simulink model "DC_5L"  (R2017b)
settings: Solver=VariableStepAuto  StartTime=0.0  StopTime=2  MaxStep=1e-4  RelTol=1e-3
libraries: powerlib x69, peTransforms x1, powerlib_meascontrol x1
settings Model: Creator=alfonso  LastModifiedBy=alfonso

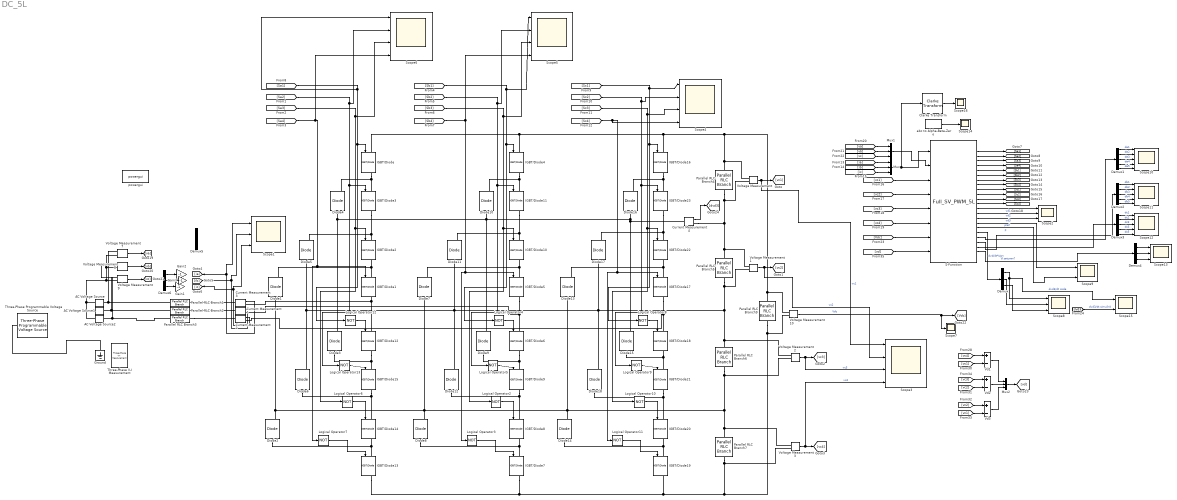
== system DC_5L ==
  AC Voltage Source : powerlib/Electrical Sources/AC Voltage Source  Amplitude=230*sqrt(2)  Phase=0  Frequency=50  SampleTime=0  Measurements=None  BusType=swing  Pref=10e3  Qref=0  Qmin=-inf  Qmax=+inf
  AC Voltage Source1 : powerlib/Electrical Sources/AC Voltage Source  Amplitude=230*sqrt(2)  Phase=120  Frequency=50  SampleTime=0  Measurements=None  BusType=swing  Pref=10e3  Qref=0  Qmin=-inf  Qmax=+inf
  AC Voltage Source2 : powerlib/Electrical Sources/AC Voltage Source  Amplitude=230*sqrt(2)  Phase=240  Frequency=50  SampleTime=0  Measurements=None  BusType=swing  Pref=10e3  Qref=0  Qmin=-inf  Qmax=+inf
  Clarke Transform : peTransforms/Clarke Transform  PowerInvariant=on
  Current Measurement{1..4} (4 alike) : powerlib/Measurements/Current Measurement  PhasorSimulation=off  OutputType=Complex  PSBequivalent=0
  Demux{,4..6} (4 alike) : Demux  Outputs=3
  Demux1 : Demux  Outputs=5
  Demux2 : Demux  Outputs=5
  Demux3 : Demux  Outputs=5
  Diode{1..18} (18 alike) : powerlib/Power Electronics/Diode  Ron=0.001  Lon=0  Vf=0.8  IC=0  UseSnubber=0  Rs=500  Cs=250e-9  Measurements=on
  Gain1 : Gain  Gain=-1
  Gain2 : Gain  Gain=-1
  Gain3 : Gain  Gain=-1
  Ground : powerlib/Elements/Ground  LConnTagsString=a
  IGBT/Diode{,1..23} (24 alike) : powerlib/Power Electronics/IGBT//Diode  Ron=1e-3  Rs=1e5  Cs=inf  Measurements=on
  Logical Operator{2..13} (12 alike) : Logic  Operator=NOT  AllPortsSameDT=off  OutDataTypeStr=boolean
  Mux : Mux  Inputs=3
  Mux1 : Mux  Inputs=3
  Mux2 : Mux  Inputs=3
  Parallel RLC Branch1 : powerlib/Elements/Parallel RLC Branch  LConnTagsString=a  RConnTagsString=__new0  BranchType=L  Resistance=0  Inductance=2e-3  SetiL0=off  InitialCurrent=0  Capacitance=7e-3  Setx0=off  InitialVoltage=0  Measurements=None
  Parallel RLC Branch2 : powerlib/Elements/Parallel RLC Branch  LConnTagsString=a  RConnTagsString=__new0  BranchType=L  Resistance=0  Inductance=2e-3  SetiL0=off  InitialCurrent=0  Capacitance=7e-3  Setx0=off  InitialVoltage=0  Measurements=None
  Parallel RLC Branch3 : powerlib/Elements/Parallel RLC Branch  LConnTagsString=a  RConnTagsString=__new0  BranchType=L  Resistance=0  Inductance=2e-3  SetiL0=off  InitialCurrent=0  Capacitance=7e-3  Setx0=off  InitialVoltage=0  Measurements=None
  Parallel RLC Branch{4..7} (4 alike) : powerlib/Elements/Parallel RLC Branch  LConnTagsString=a  RConnTagsString=__new0  BranchType=C  Resistance=0  Inductance=0  SetiL0=off  InitialCurrent=0  Capacitance=3.3e-3  Setx0=off  InitialVoltage=0  Measurements=None
  Parallel RLC Branch9 : powerlib/Elements/Parallel RLC Branch  LConnTagsString=a  RConnTagsString=__new0  BranchType=R  Resistance=300  Inductance=0  SetiL0=off  InitialCurrent=0  Capacitance=1e-3  Setx0=off  InitialVoltage=0  Measurements=None
  S-Function : S-Function  FunctionName=Full_SV_PWM_5L  SFunctionDeploymentMode=off  EnableBusSupport=off
  Scope{1..2,8,13} (4 alike) : Scope  NumInputPorts=3
  Scope10 : Scope  NumInputPorts=5
  Scope11 : Scope  NumInputPorts=5
  Scope12 : Scope  NumInputPorts=5
  Scope14 : Scope
  Scope15 : Scope  NumInputPorts=2
  Scope16 : Scope
  Scope{3..6} (4 alike) : Scope  NumInputPorts=4
  Scope7 : Scope
  Scope9 : Scope  NumInputPorts=2
  Three-Phase Programmable Voltage Source : powerlib/Electrical Sources/Three-Phase Programmable Voltage Source  PositiveSequence="[230*sqrt(3)  0 50]"  VariationEntity=None  VariationType=Table of time-amplitude pairs  VariationTypeAlt=Step  VariationStep=0.5  VariationRate=10  VariationMagnitude=0.3  VariationFrequency=2  VariationTiming=[1 2]  VariationPhaseA=off  Amplitudes=[1 0.8 1.2 1.0]  TimeValues=[0 0.1 0.15 0.2]  HarmonicGeneration=off  HarmonicA=[3 0.2 -25 0]  HarmonicB=[2 0.15 35 2]  Timing="[0.05  3]"  BusType=swing  Pref=0  Qref=0  Qmin=-inf  Qmax=inf
  Three-Phase V-I Measurement : powerlib/Measurements/Three-Phase V-I Measurement  VoltageMeasurement=phase-to-ground  SetLabelV=off  LabelV=Vabc  Vpu=off  VpuLL=off  CurrentMeasurement=yes  SetLabelI=off  LabelI=Iabc  Ipu=off  Pbase=100e6  Vbase=500e3  OutputType=Complex  PhasorSimulation=off  PSBequivalent=0
  Vd1 : Sum  Inputs=+-
  Vd2 : Sum  Inputs=+-
  Vd3 : Sum  Inputs=+-
  Voltage Measurement{,1..3,7..10} (8 alike) : powerlib/Measurements/Voltage Measurement  PhasorSimulation=off  OutputType=Complex  PSBequivalent=0
  abc to Alpha-Beta-Zero : powerlib_meascontrol/Transformations/abc to Alpha-Beta-Zero
      settings: SourceProductName=Simscape Power Systems
  powergui : powerlib/powergui  Priority=1  SimulationMode=Continuous  SampleTime=50e-6  frequency=60  Iterations=50  frequencyindice=50  Pbase=100e6  ErrMax=1e-4  UnitsV=kV  UnitsW=MW  buscounter=0  FunctionMessages=off  echomessages=off  EnableUseOfTLC=off  CurrentSourceSwitches=off  DisableSnubberDevices=off  DisableRonSwitches=off  DisableVfSwitches=off  DisplayEquations=off  SolverType=Tustin/Backward Euler (TBE)  Interpol=off  ExternalGateDelay=off  methode=off  Ts=100  x0status=blocks  SPID=on  SwTol=0  HookPort=off  RestoreLinks=warning  ResistiveCurrentMeasurement=off  Frange=[0:2:500]  Ylog=off  Xlog=on  ShowGrid=off  save=off  variable=ZData  structure=0  ZoomFFT=off  StartTime=0.0  cycles=1  DisplayStyle=1  fundamental=60  FreqAxis=off  MaxFrequency=1000  frequencyindicesteady=1  RmsSteady=1  display=off
  wires:
  [Sc2] -> Scope4/2, IGBT/Diode23/1, Logical Operator9/1
  [Sc3] -> Scope4/3, Logical Operator10/1, IGBT/Diode22/1
  [Sc4] -> Scope4/4, IGBT/Diode17/1, Logical Operator11/1
  Logical Operator11/1 -> IGBT/Diode19/1
  Logical Operator10/1 -> IGBT/Diode20/1
  Logical Operator9/1 -> IGBT/Diode21/1
  Logical Operator8/1 -> IGBT/Diode18/1
  Logical Operator3/1 -> IGBT/Diode7/1
  Logical Operator4/1 -> IGBT/Diode6/1
  Logical Operator5/1 -> IGBT/Diode9/1
  Logical Operator2/1 -> IGBT/Diode8/1
  Logical Operator6/1 -> IGBT/Diode14/1
  Logical Operator7/1 -> IGBT/Diode13/1
  Logical Operator13/1 -> IGBT/Diode15/1
  Logical Operator12/1 -> IGBT/Diode12/1
  Voltage Measurement/1 -> Scope3/1, [vc1]  "vc1"
  Voltage Measurement1/1 -> Scope3/2, [vc2]  "vc2"
  Voltage Measurement2/1 -> Scope3/3, [vc3]  "vc3"
  Voltage Measurement3/1 -> Scope3/4, [vc4]  "vc4"
  [ia] -> Mux/1
  [ib] -> Mux/2
  [ic] -> Mux/3
  S-Function/12 -> [Sc4]
  S-Function/11 -> [Sc3]
  S-Function/10 -> [Sc2]
  S-Function/9 -> [Sc1]
  S-Function/8 -> [Sb4]
  S-Function/7 -> [Sb3]
  S-Function/6 -> [Sb2]
  S-Function/5 -> [Sb1]
  S-Function/4 -> [Sa4]
  S-Function/1 -> [Sa1]
  S-Function/2 -> [Sa2]
  S-Function/3 -> [Sa3]
  S-Function/13 -> Scope2/1  "vd1"
  S-Function/14 -> Scope2/2  "vd2"
  S-Function/15 -> Scope2/3  "vd3"
  [Sc1] -> Scope4/1, IGBT/Diode16/1, Logical Operator8/1
  S-Function/16 -> Scope9/1  "pref"
  [vc4] -> S-Function/6
  [vc3] -> S-Function/5
  [vc2] -> S-Function/4
  [vc1] -> S-Function/3
  [vc] -> Mux1/3
  [vb] -> Mux1/2
  [va] -> Mux1/1
  [Sb2] -> Scope5/2, IGBT/Diode11/1, Logical Operator5/1
  [Sb3] -> Scope5/3, IGBT/Diode10/1, Logical Operator2/1
  [Sb1] -> Scope5/1, IGBT/Diode4/1, Logical Operator4/1
  [Sb4] -> Logical Operator3/1, IGBT/Diode5/1, Scope5/4
  [Sa3] -> Scope6/3, IGBT/Diode2/1, Logical Operator6/1
  [Sa2] -> Scope6/2, IGBT/Diode3/1, Logical Operator13/1
  [Sa4] -> Scope6/4, Logical Operator7/1, IGBT/Diode1/1
  [Sa1] -> Scope6/1, IGBT/Diode/1, Logical Operator12/1
  Voltage Measurement10/1 -> Scope7/1, [Vdc]  "Vdc"
  Current Measurement3/1 -> [ia], Scope1/1
  Current Measurement2/1 -> [ic], Scope1/3
  [Vdc] -> S-Function/7
  Mux1/1 -> S-Function/2
  S-Function/17 -> Scope9/2  "p"
  S-Function/18 -> Demux/1  "dvd/dt*sign"
  Demux/1 -> Scope15/1, Scope8/1  "dvd3/dt code"
  Demux/2 -> Scope8/2
  Demux/3 -> Scope8/3
  S-Function/22 -> Demux4/1  "d saturan?"
  S-Function/21 -> Demux3/1
  S-Function/20 -> Demux2/1
  S-Function/19 -> Demux1/1
  Demux1/1 -> Scope10/1  "da1"
  Demux1/2 -> Scope10/2  "da2"
  Demux1/3 -> Scope10/3  "da3"
  Demux1/4 -> Scope10/4  "da4"
  Demux2/4 -> Scope11/4  "db4"
  Demux2/2 -> Scope11/2  "db2"
  Demux2/3 -> Scope11/3  "db3"
  Demux2/1 -> Scope11/1  "db1"
  Demux3/4 -> Scope12/4  "dc3"
  Demux3/2 -> Scope12/2  "dc2"
  Demux3/3 -> Scope12/3  "dc3"
  Demux3/1 -> Scope12/1  "dc1"
  Demux4/1 -> Scope13/1
  Demux4/2 -> Scope13/2
  Demux4/3 -> Scope13/3
  Demux3/5 -> Scope12/5  "dc5"
  Demux2/5 -> Scope11/5  "db5"
  Demux1/5 -> Scope10/5  "da5"
  Demux6/1 -> Gain2/1
  Demux6/2 -> Gain3/1
  Demux6/3 -> Gain1/1
  Current Measurement1/1 -> [ib], Scope1/2
  Voltage Measurement7/1 -> [va]
  Voltage Measurement9/1 -> [vc]
  Voltage Measurement8/1 -> [vb]
  abc to Alpha-Beta-Zero/1 -> Scope14/1
  Clarke Transform/1 -> Scope16/1
  Mux/1 -> S-Function/1, Clarke Transform/1
  Vd2/1 -> Mux2/2
  [vc1] -> Vd1/2
  Vd1/1 -> Mux2/1
  [vc2] -> Vd2/2
  [vc2] -> Vd3/1
  Vd3/1 -> Mux2/3
  [vc4] -> Vd1/1
  [vc3] -> Vd2/1
  [vc1] -> Vd3/2
  Mux2/1 -> [vd]
  [vd] -> S-Function/8
  Current Measurement4/1 -> [dvd3]
  [dvd3] -> Scope15/2  "dvd3/dt simulink"
  connections:
  IGBT/Diode/RConn1 -- Diode4/RConn1 -- IGBT/Diode3/LConn1
  IGBT/Diode1/LConn1 -- Diode1/RConn1 -- IGBT/Diode2/RConn1
  IGBT/Diode3/RConn1 -- Diode5/RConn1 -- IGBT/Diode2/LConn1
  IGBT/Diode15/RConn1 -- IGBT/Diode14/LConn1 -- Diode6/LConn1
  IGBT/Diode13/LConn1 -- Diode2/LConn1 -- IGBT/Diode14/RConn1
  IGBT/Diode12/RConn1 -- Diode3/LConn1 -- IGBT/Diode15/LConn1
  IGBT/Diode1/RConn1 -- Current Measurement3/RConn1 -- IGBT/Diode12/LConn1
  Diode15/RConn1 -- Diode16/LConn1 -- Diode4/LConn1 -- Diode3/RConn1 -- Diode10/LConn1 -- Diode9/RConn1 -- Current Measurement4/LConn1
  Parallel RLC Branch5/RConn1 -- Voltage Measurement1/LConn2 -- Diode5/LConn1 -- Diode6/RConn1 -- Diode11/LConn1 -- Diode12/RConn1 -- Diode18/RConn1 -- Diode17/LConn1 -- Voltage Measurement2/LConn1 -- Parallel RLC Branch6/LConn1
  IGBT/Diode11/RConn1 -- Diode11/RConn1 -- IGBT/Diode10/LConn1
  IGBT/Diode5/LConn1 -- Diode7/RConn1 -- IGBT/Diode10/RConn1
  IGBT/Diode9/RConn1 -- IGBT/Diode8/LConn1 -- Diode12/LConn1
  IGBT/Diode7/LConn1 -- Diode8/LConn1 -- IGBT/Diode8/RConn1
  IGBT/Diode4/RConn1 -- Diode10/RConn1 -- IGBT/Diode11/LConn1
  IGBT/Diode6/RConn1 -- Diode9/LConn1 -- IGBT/Diode9/LConn1
  IGBT/Diode5/RConn1 -- Current Measurement1/RConn1 -- IGBT/Diode6/LConn1
  IGBT/Diode23/RConn1 -- Diode17/RConn1 -- IGBT/Diode22/LConn1
  IGBT/Diode17/LConn1 -- Diode13/RConn1 -- IGBT/Diode22/RConn1
  IGBT/Diode21/RConn1 -- IGBT/Diode20/LConn1 -- Diode18/LConn1
  IGBT/Diode19/LConn1 -- Diode14/LConn1 -- IGBT/Diode20/RConn1
  IGBT/Diode16/RConn1 -- Diode16/RConn1 -- IGBT/Diode23/LConn1
  IGBT/Diode18/RConn1 -- Diode15/LConn1 -- IGBT/Diode21/LConn1
  IGBT/Diode17/RConn1 -- Current Measurement2/RConn1 -- IGBT/Diode18/LConn1
  Diode2/RConn1 -- Voltage Measurement2/LConn2 -- Parallel RLC Branch6/RConn1 -- Voltage Measurement3/LConn1 -- Parallel RLC Branch7/LConn1 -- Diode14/RConn1 -- Diode13/LConn1 -- Diode7/LConn1 -- Diode8/RConn1 -- Diode1/LConn1
  Parallel RLC Branch7/RConn1 -- Voltage Measurement3/LConn2 -- Voltage Measurement10/LConn2 -- Parallel RLC Branch9/RConn1 -- IGBT/Diode13/RConn1 -- IGBT/Diode7/RConn1 -- IGBT/Diode19/RConn1
  Parallel RLC Branch3/LConn1 -- Current Measurement2/LConn1
  Parallel RLC Branch2/LConn1 -- Current Measurement1/LConn1
  Parallel RLC Branch1/LConn1 -- Current Measurement3/LConn1
  IGBT/Diode/LConn1 -- Voltage Measurement10/LConn1 -- Parallel RLC Branch9/LConn1 -- Voltage Measurement/LConn1 -- Parallel RLC Branch4/LConn1 -- IGBT/Diode16/LConn1 -- IGBT/Diode4/LConn1
  AC Voltage Source/LConn1 -- Voltage Measurement7/LConn2 -- Voltage Measurement8/LConn2 -- Voltage Measurement9/LConn2 -- AC Voltage Source2/LConn1 -- AC Voltage Source1/LConn1
  Parallel RLC Branch1/RConn1 -- Voltage Measurement7/LConn1 -- AC Voltage Source/RConn1
  Parallel RLC Branch2/RConn1 -- Voltage Measurement8/LConn1 -- AC Voltage Source1/RConn1
  Parallel RLC Branch3/RConn1 -- Voltage Measurement9/LConn1 -- AC Voltage Source2/RConn1
  Ground/LConn1 -- Three-Phase Programmable Voltage Source/LConn1
  Voltage Measurement1/LConn1 -- Parallel RLC Branch4/RConn1 -- Voltage Measurement/LConn2 -- Current Measurement4/RConn1 -- Parallel RLC Branch5/LConn1
